simulink model "exampleTRYradiationFilter"  (Simulink 8.2)
settings: Solver=VariableStepDiscrete  StartTime=90*24*3600  StopTime=95*24*3600  MaxStep=60  RelTol=1e-3
libraries: carnot x2
settings Model: Creator=drhf  LastModifiedBy=drhf
settings DataIOCC: SignalLoggingSaveFormat=Dataset
settings DebuggingCC: FcnCallInpInsideContextMsg=EnableAllAsError

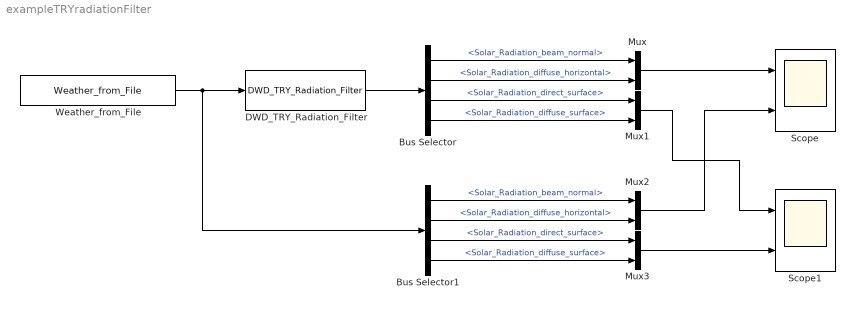
== system exampleTRYradiationFilter ==
  Bus Selector : BusSelector  OutputSignals=Solar_Radiation_beam_normal,Solar_Radiation_diffuse_horizontal,Solar_Radiation_direct_surface,Solar_Radiation_diffuse_surface
  Bus Selector1 : BusSelector  OutputSignals=Solar_Radiation_beam_normal,Solar_Radiation_diffuse_horizontal,Solar_Radiation_direct_surface,Solar_Radiation_diffuse_surface
  DWD_TRY_Radiation_Filter : carnot/Weather/DWD_TRY_Radiation_Filter  f=5
  Mux{,1..3} (4 alike) : Mux  Inputs=2
  Scope : Scope  NumInputPorts=2
      settings: YMin=-5~-5  YMax=5~5
  Scope1 : Scope  NumInputPorts=2
      settings: YMin=-5~-5  YMax=5~5
  Weather_from_File : carnot/Weather/Weather_from_File  file=DE_TRY2010_09_averageYear  ext=.mat
  wires:
  Bus Selector/1 -> Mux/1  "<Solar_Radiation_beam_normal>"
  Bus Selector/2 -> Mux/2  "<Solar_Radiation_diffuse_horizontal>"
  Bus Selector/3 -> Mux1/1  "<Solar_Radiation_direct_surface>"
  Bus Selector/4 -> Mux1/2  "<Solar_Radiation_diffuse_surface>"
  Mux/1 -> Scope/1
  DWD_TRY_Radiation_Filter/1 -> Bus Selector/1
  Bus Selector1/1 -> Mux2/1  "<Solar_Radiation_beam_normal>"
  Bus Selector1/2 -> Mux2/2  "<Solar_Radiation_diffuse_horizontal>"
  Bus Selector1/3 -> Mux3/1  "<Solar_Radiation_direct_surface>"
  Bus Selector1/4 -> Mux3/2  "<Solar_Radiation_diffuse_surface>"
  Weather_from_File/1 -> DWD_TRY_Radiation_Filter/1, Bus Selector1/1
  Mux2/1 -> Scope/2
  Mux1/1 -> Scope1/1
  Mux3/1 -> Scope1/2
